simulink model "AUV_ControlsPreliminary"  (R2020b)
settings: Solver=ode23t  StartTime=0.0  StopTime=300  MaxStep=0.01  RelTol=1e-3  EnableMultiTasking=on
PreLoadFcn:
  | AUV_VehicleParameters;
  | Vehicle.Body.markeropacity = 0;
model workspace: external: MATLAB File AUV_DataFile_ORIG.m (data not in the file)
undefined symbols (not defined in the file or in its folder): Environment, Multibody, Newton, Raphson, smiData, X, x, Y, y, Z
libraries: sm_lib x3123, nesl_utility x51, sharedutil x8, pid_lib x6, AUVCustomPrimitives_Lib x4, shared6dof x1, aerolibasang x1, aerolibadyn x1, SignalEditorBlockLib x1
(part 2 of 62)

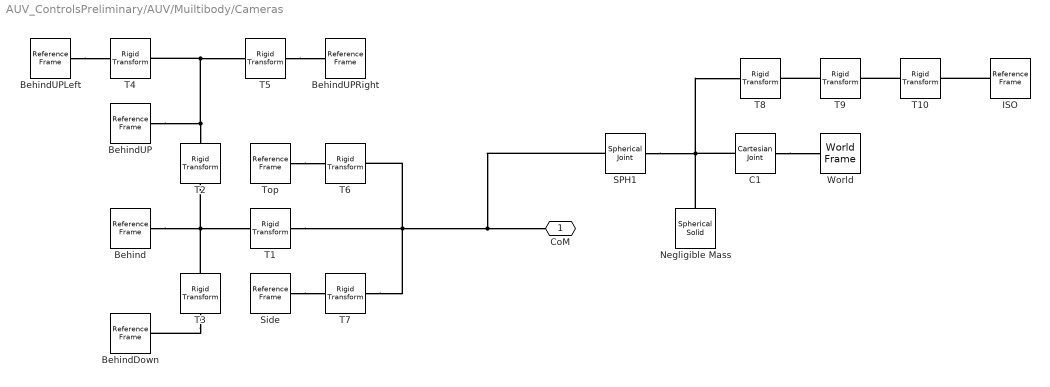
== system AUV_ControlsPreliminary/AUV/Muiltibody/Cameras ==
  Behind : sm_lib/Frames and Transforms/Reference Frame
  BehindDown : sm_lib/Frames and Transforms/Reference Frame
  BehindUP : sm_lib/Frames and Transforms/Reference Frame
  BehindUPLeft : sm_lib/Frames and Transforms/Reference Frame
  BehindUPRight : sm_lib/Frames and Transforms/Reference Frame
  C1 : sm_lib/Joints/Cartesian Joint  JointMode=Normal  SenseConstraintForce=off  SenseConstraintForceX=off  SenseConstraintForceY=off  SenseConstraintForceZ=off  SenseConstraintTorque=off  SenseConstraintTorqueX=off  SenseConstraintTorqueY=off  SenseConstraintTorqueZ=off  SenseTotalForce=off  SenseTotalForceX=off  SenseTotalForceY=off  SenseTotalForceZ=off  SenseTotalTorque=off  SenseTotalTorqueX=off  SenseTotalTorqueY=off  SenseTotalTorqueZ=off  CompositeWrenchDir=FollowerOnBase  CompositeWrenchFrame=BaseFrame  PxEquilibriumPosition=0  PxEquilibriumPositionUnits=m  PxSpringStiffness=0  PxSpringStiffnessUnits=N/m  PxDampingCoefficient=0  PxDampingCoefficientUnits=N/(m/s)  PxTorqueActuationMode=NoTorque  PxMotionActuationMode=ComputedMotion  PxSensePosition=off  PxSenseVelocity=off  PxSenseAcceleration=off  PxSenseTorqueForce=off  PxSenseLowerLimitTorqueForce=off  PxSenseUpperLimitTorqueForce=off  PxLowerLimitSpecify=off  PxLowerLimitBound=-1  PxLowerLimitBoundUnits=m  PxLowerLimitStiffness=1e6  PxLowerLimitStiffnessUnits=N/m  PxLowerLimitDamping=1e3  PxLowerLimitDampingUnits=N/(m/s)  PxLowerLimitTransitionRegionWidth=1e-4  PxLowerLimitTransitionRegionWidthUnits=m  PxUpperLimitSpecify=off  PxUpperLimitBound=1  PxUpperLimitBoundUnits=m  PxUpperLimitStiffness=1e6  PxUpperLimitStiffnessUnits=N/m  PxUpperLimitDamping=1e3  PxUpperLimitDampingUnits=N/(m/s)  PxUpperLimitTransitionRegionWidth=1e-4  PxUpperLimitTransitionRegionWidthUnits=m  PxPositionTargetSpecify=off  PxPositionTargetPriority=High  PxPositionTargetValue=0  PxPositionTargetValueUnits=m  PxVelocityTargetSpecify=off  PxVelocityTargetPriority=High  PxVelocityTargetValue=0  PxVelocityTargetValueUnits=m/s  PyEquilibriumPosition=0  PyEquilibriumPositionUnits=m  PySpringStiffness=0  PySpringStiffnessUnits=N/m  PyDampingCoefficient=0  PyDampingCoefficientUnits=N/(m/s)  PyTorqueActuationMode=NoTorque  PyMotionActuationMode=ComputedMotion  PySensePosition=off  PySenseVelocity=off  PySenseAcceleration=off  PySenseTorqueForce=off  PySenseLowerLimitTorqueForce=off  PySenseUpperLimitTorqueForce=off  PyLowerLimitSpecify=off  PyLowerLimitBound=-1  PyLowerLimitBoundUnits=m  PyLowerLimitStiffness=1e6  PyLowerLimitStiffnessUnits=N/m  PyLowerLimitDamping=1e3  PyLowerLimitDampingUnits=N/(m/s)  PyLowerLimitTransitionRegionWidth=1e-4  PyLowerLimitTransitionRegionWidthUnits=m  PyUpperLimitSpecify=off  PyUpperLimitBound=1  PyUpperLimitBoundUnits=m  PyUpperLimitStiffness=1e6  PyUpperLimitStiffnessUnits=N/m  PyUpperLimitDamping=1e3  PyUpperLimitDampingUnits=N/(m/s)  PyUpperLimitTransitionRegionWidth=1e-4  PyUpperLimitTransitionRegionWidthUnits=m  PyPositionTargetSpecify=off  PyPositionTargetPriority=High  PyPositionTargetValue=0  PyPositionTargetValueUnits=m  PyVelocityTargetSpecify=off  PyVelocityTargetPriority=High  PyVelocityTargetValue=0  PyVelocityTargetValueUnits=m/s  PzEquilibriumPosition=0  PzEquilibriumPositionUnits=m  PzSpringStiffness=0  PzSpringStiffnessUnits=N/m  PzDampingCoefficient=0  PzDampingCoefficientUnits=N/(m/s)  PzTorqueActuationMode=NoTorque  PzMotionActuationMode=ComputedMotion  PzSensePosition=off  PzSenseVelocity=off  PzSenseAcceleration=off  PzSenseTorqueForce=off  PzSenseLowerLimitTorqueForce=off  PzSenseUpperLimitTorqueForce=off  PzLowerLimitSpecify=off  PzLowerLimitBound=-1  PzLowerLimitBoundUnits=m  PzLowerLimitStiffness=1e6  PzLowerLimitStiffnessUnits=N/m  PzLowerLimitDamping=1e3  PzLowerLimitDampingUnits=N/(m/s)  PzLowerLimitTransitionRegionWidth=1e-4  PzLowerLimitTransitionRegionWidthUnits=m  PzUpperLimitSpecify=off  PzUpperLimitBound=1  PzUpperLimitBoundUnits=m  PzUpperLimitStiffness=1e6  PzUpperLimitStiffnessUnits=N/m  PzUpperLimitDamping=1e3  PzUpperLimitDampingUnits=N/(m/s)  PzUpperLimitTransitionRegionWidth=1e-4  PzUpperLimitTransitionRegionWidthUnits=m  PzPositionTargetSpecify=off  PzPositionTargetPriority=High  PzPositionTargetValue=0  PzPositionTargetValueUnits=m  PzVelocityTargetSpecify=off  PzVelocityTargetPriority=High  PzVelocityTargetValue=0  PzVelocityTargetValueUnits=m/s
  ISO : sm_lib/Frames and Transforms/Reference Frame
  Negligible Mass : sm_lib/Body Elements/Spherical Solid  GraphicAmbientColor=[0.15 0.15 0.15 1.0]  BasedOnType=Mass  CenterOfMass=[0 0 0]  CenterOfMassUnits=m  GraphicDiffuseColor=[0.5 0.5 0.5]  Density=1000  DensityUnits=kg/m^3  DoExposeReferenceFrame=on  GraphicEmissiveColor=[0.0 0.0 0.0 1.0]  ExportEntireGeometry=off  SerializedExposedGeometries=<ExposedGeometries/>  SerializedFrames=<Frames/>  MarkerShape=Sphere  MarkerSize=10  GraphicType=FromGeometry  InertiaType=CalculateFromGeometry  Mass=1e-6  MassUnits=kg  MomentsOfInertia=[1 1 1]  MomentsOfInertiaUnits=kg*m^2  GraphicOpacity=0  ProductsOfInertia=[0 0 0]  ProductsOfInertiaUnits=kg*m^2  GraphicShininess=75  GraphicSpecularColor=[0.5 0.5 0.5 1.0]  SphereRadius=1e-3  SphereRadiusUnits=m  GraphicVisPropType=SimpleVisualProperties
  SPH1 : sm_lib/Joints/Spherical Joint  JointMode=Normal  SenseConstraintForce=off  SenseConstraintForceX=off  SenseConstraintForceY=off  SenseConstraintForceZ=off  SenseConstraintTorque=off  SenseConstraintTorqueX=off  SenseConstraintTorqueY=off  SenseConstraintTorqueZ=off  SenseTotalForce=off  SenseTotalForceX=off  SenseTotalForceY=off  SenseTotalForceZ=off  SenseTotalTorque=off  SenseTotalTorqueX=off  SenseTotalTorqueY=off  SenseTotalTorqueZ=off  CompositeWrenchDir=FollowerOnBase  CompositeWrenchFrame=BaseFrame  DefPosRotationMethod=None  DefPosRotationAngleUnits=deg  DefPosRotationStandardAxis=+Z  DefPosRotationAngle=0.0  DefPosRotationArbitraryAxis=[0 0 1]  DefPosFollAlignAxisA=+X  DefPosBaseAlignAxisA=+Y  DefPosFollAlignAxisB=+Y  DefPosBaseAlignAxisB=+Z  DefPosRotationSequenceAxes=FollowerAxes  DefPosRotationSequence=XYX  DefPosRotationSequenceAngles=[0 0 0]  DefPosRotationSequenceAnglesUnits=deg  DefPosRotationMatrix=[1 0 0; 0 1 0; 0 0 1]  EqPosRotationMethod=None  EqPosRotationAngleUnits=deg  EqPosRotationStandardAxis=+Z  EqPosRotationAngle=0.0  EqPosRotationArbitraryAxis=[0 0 1]  EqPosFollAlignAxisA=+X  EqPosBaseAlignAxisA=+Y  EqPosFollAlignAxisB=+Y  EqPosBaseAlignAxisB=+Z  EqPosRotationSequenceAxes=FollowerAxes  EqPosRotationSequence=XYX  EqPosRotationSequenceAngles=[0 0 0]  EqPosRotationSequenceAnglesUnits=deg  EqPosRotationMatrix=[1 0 0; 0 1 0; 0 0 1]  SpringStiffness=0  SpringStiffnessUnits=N*m/deg  DampingCoefficient=0  DampingCoefficientUnits=N*m/(deg/s)  ActuateTorqueX=off  ActuateTorqueY=off  ActuateTorqueZ=off  ActuateTorque=off  TorqueActuationMode=NoTorque  MotionActuationMode=ComputedMotion  ActuationFrame=BaseFrame  SensePosition=off  SenseVelocityX=off  SenseVelocityY=off  SenseVelocityZ=off  SenseVelocity=off  SenseAccelerationX=off  SenseAccelerationY=off  SenseAccelerationZ=off  SenseAcceleration=off  SenseTorqueX=off  SenseTorqueY=off  SenseTorqueZ=off  SenseTorqueForce=off  SenseLowerLimitTorqueMag=off  SenseUpperLimitTorqueMag=off  SensingFrame=BaseFrame  LowerLimitSpecify=off  LowerLimitBound=15  LowerLimitBoundUnits=deg  LowerLimitStiffness=1e4  LowerLimitStiffnessUnits=N*m/deg  LowerLimitDamping=10  LowerLimitDampingUnits=N*m/(deg/s)  LowerLimitTransitionRegionWidth=0.1  LowerLimitTransitionRegionWidthUnits=deg  UpperLimitSpecify=off  UpperLimitBound=45  UpperLimitBoundUnits=deg  UpperLimitStiffness=1e4  UpperLimitStiffnessUnits=N*m/deg  UpperLimitDamping=10  UpperLimitDampingUnits=N*m/(deg/s)  UpperLimitTransitionRegionWidth=0.1  UpperLimitTransitionRegionWidthUnits=deg  PositionTargetRotationMethod=None  PositionTargetRotationAngleUnits=deg  PositionTargetRotationStandardAxis=+Z  PositionTargetRotationAngle=0.0  PositionTargetRotationArbitraryAxis=[0 0 1]  PositionTargetFollAlignAxisA=+X  PositionTargetBaseAlignAxisA=+Y  PositionTargetFollAlignAxisB=+Y  PositionTargetBaseAlignAxisB=+Z  PositionTargetRotationSequenceAxes=FollowerAxes  PositionTargetRotationSequence=XYX  PositionTargetRotationSequenceAngles=[0 0 0]  PositionTargetRotationSequenceAnglesUnits=deg  PositionTargetRotationMatrix=[1 0 0; 0 1 0; 0 0 1]  PositionTargetSpecify=off  PositionTargetPriority=High  VelocityTargetValue=[0 0 0]  VelocityTargetValueUnits=deg/s  VelocityTargetSpecify=off  VelocityTargetPriority=High  VelocityTargetInFollowerFrame=on
  Side : sm_lib/Frames and Transforms/Reference Frame
  T1 : sm_lib/Frames and Transforms/Rigid Transform  TranslationMethod=Cartesian  TranslationStandardOffset=0  TranslationLengthUnit=m  TranslationStandardAxis=+Z  TranslationCartesianOffset=[-3 0 0]  TranslationROffset=0  TranslationROffsetUnits=m  TranslationZOffset=0  TranslationZOffsetUnits=m  TranslationThetaOffset=0  TranslationThetaOffsetUnits=deg  RotationMethod=None  RotationAngleUnits=deg  RotationStandardAxis=+Z  RotationAngle=0.0  RotationArbitraryAxis=[0 0 1]  FollAlignAxisA=+X  BaseAlignAxisA=+Y  FollAlignAxisB=+Y  BaseAlignAxisB=+Z  RotationSequenceAxes=FollowerAxes  RotationSequence=XYX  RotationSequenceAngles=[0 0 0]  RotationSequenceAnglesUnits=deg  RotationMatrix=[1 0 0; 0 1 0; 0 0 1]
  T10 : sm_lib/Frames and Transforms/Rigid Transform  TranslationMethod=Cartesian  TranslationStandardOffset=0  TranslationLengthUnit=m  TranslationStandardAxis=+Z  TranslationCartesianOffset=[0 -1.5 0]  TranslationROffset=0  TranslationROffsetUnits=m  TranslationZOffset=0  TranslationZOffsetUnits=m  TranslationThetaOffset=0  TranslationThetaOffsetUnits=deg  RotationMethod=None  RotationAngleUnits=deg  RotationStandardAxis=+Z  RotationAngle=0.0  RotationArbitraryAxis=[0 0 1]  FollAlignAxisA=+X  BaseAlignAxisA=+Y  FollAlignAxisB=+Y  BaseAlignAxisB=+Z  RotationSequenceAxes=FollowerAxes  RotationSequence=XYX  RotationSequenceAngles=[0 0 0]  RotationSequenceAnglesUnits=deg  RotationMatrix=[1 0 0; 0 1 0; 0 0 1]
  T2 : sm_lib/Frames and Transforms/Rigid Transform  TranslationMethod=Cartesian  TranslationStandardOffset=0  TranslationLengthUnit=m  TranslationStandardAxis=+Z  TranslationCartesianOffset=[0 0 -3]  TranslationROffset=0  TranslationROffsetUnits=m  TranslationZOffset=0  TranslationZOffsetUnits=m  TranslationThetaOffset=0  TranslationThetaOffsetUnits=deg  RotationMethod=None  RotationAngleUnits=deg  RotationStandardAxis=+Z  RotationAngle=0.0  RotationArbitraryAxis=[0 0 1]  FollAlignAxisA=+X  BaseAlignAxisA=+Y  FollAlignAxisB=+Y  BaseAlignAxisB=+Z  RotationSequenceAxes=FollowerAxes  RotationSequence=XYX  RotationSequenceAngles=[0 0 0]  RotationSequenceAnglesUnits=deg  RotationMatrix=[1 0 0; 0 1 0; 0 0 1]
  T3 : sm_lib/Frames and Transforms/Rigid Transform  TranslationMethod=Cartesian  TranslationStandardOffset=0  TranslationLengthUnit=m  TranslationStandardAxis=+Z  TranslationCartesianOffset=[0 0 -3]  TranslationROffset=0  TranslationROffsetUnits=m  TranslationZOffset=0  TranslationZOffsetUnits=m  TranslationThetaOffset=0  TranslationThetaOffsetUnits=deg  RotationMethod=None  RotationAngleUnits=deg  RotationStandardAxis=+Z  RotationAngle=0.0  RotationArbitraryAxis=[0 0 1]  FollAlignAxisA=+X  BaseAlignAxisA=+Y  FollAlignAxisB=+Y  BaseAlignAxisB=+Z  RotationSequenceAxes=FollowerAxes  RotationSequence=XYX  RotationSequenceAngles=[0 0 0]  RotationSequenceAnglesUnits=deg  RotationMatrix=[1 0 0; 0 1 0; 0 0 1]
  T4 : sm_lib/Frames and Transforms/Rigid Transform  TranslationMethod=Cartesian  TranslationStandardOffset=0  TranslationLengthUnit=m  TranslationStandardAxis=+Z  TranslationCartesianOffset=[0 -2 0]  TranslationROffset=0  TranslationROffsetUnits=m  TranslationZOffset=0  TranslationZOffsetUnits=m  TranslationThetaOffset=0  TranslationThetaOffsetUnits=deg  RotationMethod=None  RotationAngleUnits=deg  RotationStandardAxis=+Z  RotationAngle=0.0  RotationArbitraryAxis=[0 0 1]  FollAlignAxisA=+X  BaseAlignAxisA=+Y  FollAlignAxisB=+Y  BaseAlignAxisB=+Z  RotationSequenceAxes=FollowerAxes  RotationSequence=XYX  RotationSequenceAngles=[0 0 0]  RotationSequenceAnglesUnits=deg  RotationMatrix=[1 0 0; 0 1 0; 0 0 1]
  T5 : sm_lib/Frames and Transforms/Rigid Transform  TranslationMethod=Cartesian  TranslationStandardOffset=0  TranslationLengthUnit=m  TranslationStandardAxis=+Z  TranslationCartesianOffset=[0 -2 0]  TranslationROffset=0  TranslationROffsetUnits=m  TranslationZOffset=0  TranslationZOffsetUnits=m  TranslationThetaOffset=0  TranslationThetaOffsetUnits=deg  RotationMethod=None  RotationAngleUnits=deg  RotationStandardAxis=+Z  RotationAngle=0.0  RotationArbitraryAxis=[0 0 1]  FollAlignAxisA=+X  BaseAlignAxisA=+Y  FollAlignAxisB=+Y  BaseAlignAxisB=+Z  RotationSequenceAxes=FollowerAxes  RotationSequence=XYX  RotationSequenceAngles=[0 0 0]  RotationSequenceAnglesUnits=deg  RotationMatrix=[1 0 0; 0 1 0; 0 0 1]
  T6 : sm_lib/Frames and Transforms/Rigid Transform  TranslationMethod=Cartesian  TranslationStandardOffset=0  TranslationLengthUnit=m  TranslationStandardAxis=+Z  TranslationCartesianOffset=[0 0 -3]  TranslationROffset=0  TranslationROffsetUnits=m  TranslationZOffset=0  TranslationZOffsetUnits=m  TranslationThetaOffset=0  TranslationThetaOffsetUnits=deg  RotationMethod=None  RotationAngleUnits=deg  RotationStandardAxis=+Z  RotationAngle=0.0  RotationArbitraryAxis=[0 0 1]  FollAlignAxisA=+X  BaseAlignAxisA=+Y  FollAlignAxisB=+Y  BaseAlignAxisB=+Z  RotationSequenceAxes=FollowerAxes  RotationSequence=XYX  RotationSequenceAngles=[0 0 0]  RotationSequenceAnglesUnits=deg  RotationMatrix=[1 0 0; 0 1 0; 0 0 1]
  T7 : sm_lib/Frames and Transforms/Rigid Transform  TranslationMethod=Cartesian  TranslationStandardOffset=0  TranslationLengthUnit=m  TranslationStandardAxis=+Z  TranslationCartesianOffset=[0 -3 0]  TranslationROffset=0  TranslationROffsetUnits=m  TranslationZOffset=0  TranslationZOffsetUnits=m  TranslationThetaOffset=0  TranslationThetaOffsetUnits=deg  RotationMethod=None  RotationAngleUnits=deg  RotationStandardAxis=+Z  RotationAngle=0.0  RotationArbitraryAxis=[0 0 1]  FollAlignAxisA=+X  BaseAlignAxisA=+Y  FollAlignAxisB=+Y  BaseAlignAxisB=+Z  RotationSequenceAxes=FollowerAxes  RotationSequence=XYX  RotationSequenceAngles=[0 0 0]  RotationSequenceAnglesUnits=deg  RotationMatrix=[1 0 0; 0 1 0; 0 0 1]
  T8 : sm_lib/Frames and Transforms/Rigid Transform  TranslationMethod=Cartesian  TranslationStandardOffset=0  TranslationLengthUnit=m  TranslationStandardAxis=+Z  TranslationCartesianOffset=[-2.5 0 0]  TranslationROffset=0  TranslationROffsetUnits=m  TranslationZOffset=0  TranslationZOffsetUnits=m  TranslationThetaOffset=0  TranslationThetaOffsetUnits=deg  RotationMethod=None  RotationAngleUnits=deg  RotationStandardAxis=+Z  RotationAngle=0.0  RotationArbitraryAxis=[0 0 1]  FollAlignAxisA=+X  BaseAlignAxisA=+Y  FollAlignAxisB=+Y  BaseAlignAxisB=+Z  RotationSequenceAxes=FollowerAxes  RotationSequence=XYX  RotationSequenceAngles=[0 0 0]  RotationSequenceAnglesUnits=deg  RotationMatrix=[1 0 0; 0 1 0; 0 0 1]
  T9 : sm_lib/Frames and Transforms/Rigid Transform  TranslationMethod=Cartesian  TranslationStandardOffset=0  TranslationLengthUnit=m  TranslationStandardAxis=+Z  TranslationCartesianOffset=[0 0 -2.5]  TranslationROffset=0  TranslationROffsetUnits=m  TranslationZOffset=0  TranslationZOffsetUnits=m  TranslationThetaOffset=0  TranslationThetaOffsetUnits=deg  RotationMethod=None  RotationAngleUnits=deg  RotationStandardAxis=+Z  RotationAngle=0.0  RotationArbitraryAxis=[0 0 1]  FollAlignAxisA=+X  BaseAlignAxisA=+Y  FollAlignAxisB=+Y  BaseAlignAxisB=+Z  RotationSequenceAxes=FollowerAxes  RotationSequence=XYX  RotationSequenceAngles=[0 0 0]  RotationSequenceAnglesUnits=deg  RotationMatrix=[1 0 0; 0 1 0; 0 0 1]
  Top : sm_lib/Frames and Transforms/Reference Frame
  World : sm_lib/Frames and Transforms/World Frame
  CoM : PMIOPort  Side=Right
  connections:
  T1/LConn1 -- T7/LConn1 -- SPH1/LConn1 -- CoM/RConn1 -- T6/LConn1
  Behind/RConn1 -- T3/RConn1 -- T2/LConn1 -- T1/RConn1
  BehindUP/RConn1 -- T2/RConn1 -- T5/RConn1 -- T4/LConn1
  T3/LConn1 -- BehindDown/RConn1
  BehindUPLeft/RConn1 -- T4/RConn1
  T5/LConn1 -- BehindUPRight/RConn1
  Top/RConn1 -- T6/RConn1
  Side/RConn1 -- T7/RConn1
  SPH1/RConn1 -- T8/LConn1 -- C1/LConn1 -- Negligible Mass/RConn1
  C1/RConn1 -- World/RConn1
  T9/LConn1 -- T8/RConn1
  T10/LConn1 -- T9/RConn1
  ISO/RConn1 -- T10/RConn1

== system AUV_ControlsPreliminary/AUV/Muiltibody/Hydro Forces & Moments ==
  Bus Element In : Inport  PortName=HydroForces  Element=Buoyancy.BForceZ
  Bus Element In1 : Inport  PortName=HydroForces  Element=LiftNDrag.LDForcesXYZ
  Bus Element In2 : Inport  PortName=HydroForces  Element=LiftNDrag.LDMomentsXYZ
  Bus Element In3 : Inport  PortName=HydroForces  Element=AddedMass.AMForcesXYZ
  Bus Element In4 : Inport  PortName=HydroForces  Element=AddedMass.AMMomentsXYZ
  Bus Element In5 : Inport  PortName=HydroForces  Element=AddedMass.CMomentsXYZ
  Bus Element In6 : Inport  PortName=HydroForces  Element=AddedMass.CForcesXYZ
  Added Mass Coriolis : Subsystem
  Added Mass Forces : Subsystem
  Buoyancy Force : Subsystem
  Lift and Drag Forces : Subsystem
  CoM : PMIOPort  Side=Right
  CoB : PMIOPort  Port=2  Side=Right
  wires:
  Bus Element In/1 -> Buoyancy Force/1(B)
  Bus Element In1/1 -> Lift and Drag Forces/1(Fxyz)
  Bus Element In2/1 -> Lift and Drag Forces/2(Mxyz)
  Bus Element In3/1 -> Added Mass Forces/1(Fxyz)
  Bus Element In4/1 -> Added Mass Forces/2(Mxyz)
  Bus Element In5/1 -> Added Mass Coriolis/2(Mxyz)
  Bus Element In6/1 -> Added Mass Coriolis/1(Fxyz)
  connections:
  CoB/RConn1 -- Buoyancy Force/RConn1
  Lift and Drag Forces/RConn1 -- Added Mass Coriolis/RConn1 -- Added Mass Forces/RConn1 -- CoM/RConn1

== system AUV_ControlsPreliminary/AUV/Muiltibody/World ==
  Mechanism Configuration : sm_lib/Utilities/Mechanism Configuration  UniformGravity=Constant  GravityVector=[0 0 Environment.gravity]  GravityVectorUnits=m/s^2  GravityUnits=m/s^2  LinearizationDelta=0.001  JointModeTransitionNonlinearIterations=2
  Sea Floor : Subsystem
  Solver Configuration : nesl_utility/Solver Configuration  PhysicalDomain=network_engine_domain  SubClassName=solver  LeftPortType=input  RightPortType=generic  Tones=[]  Harmonics=[]  SimulateNoise=off  Profile=off  UseLocalSampling=off  EnableSwitchedLinearOptims=on  FrequencyDomain=off  UseCCode=off  RelTol=0.001  AbsTol=1e-06  MinStep=1e-09  ToWorkspace=off  RevertToSquareIcSolve=off  NumHomotopyIterations=100  PhasorMode=off  PhasorModeNumHarmonics=1  DoDC=off  ResidualTolerance=1e-09  UseLocalSolver=off  LocalSolverChoice=NE_BACKWARD_EULER_ADVANCER  LocalSolverSampleTime=0.001  DoFixedCost=off  MaxNonlinIter=3  MaxModeIter=2  ComputeImpulses=off  ImpulseIterations=2  LinearAlgebra=Sparse  EquationFormulation=NE_TIME_EF  DelaysMemoryBudget=1024  AutomaticFiltering=on  FilteringTimeConstant=0.001  PartitionStorageMethod=AS_NEEDED  PartitionMemoryBudget=1024  PartitionMethod=FAST
  World Frame --> e NED : sm_lib/Frames and Transforms/World Frame
  W : PMIOPort  Side=Right
  connections:
  World Frame --> e NED/RConn1 -- W/RConn1 -- Sea Floor/LConn1 -- Mechanism Configuration/RConn1 -- Solver Configuration/RConn1

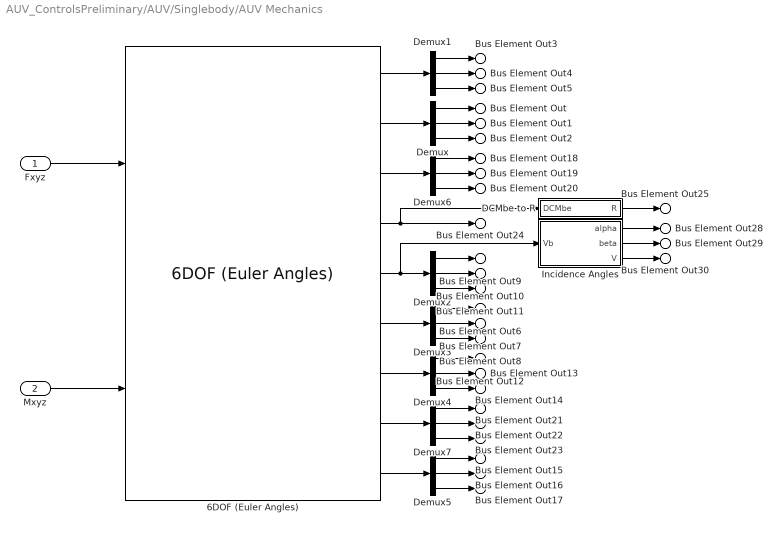
== system AUV_ControlsPreliminary/AUV/Singlebody/AUV Mechanics ==
  Fxyz : Inport
  Mxyz : Inport  Port=2
  6DOF (Euler Angles) : shared6dof/6DOF (Euler Angles)  units=Metric (MKS)  mtype=Fixed  rep=Euler Angles  xme_0=Vehicle.InitCond.position  Vm_0=Vehicle.InitCond.velocity  eul_0=Vehicle.InitCond.EulerXYZrad  pm_0=Vehicle.InitCond.rotrates  mass_0=Vehicle.Body.Full.mass  mass_e=0.5  mass_f=2.0  inertia=Vehicle.Body.Full.Inertia  inertia_e=eye(3)  inertia_f=2*eye(3)  k_quat=1.0  vre_flag=on  abi_flag=on  aMode=0  xme_statename=''  Vm_statename=''  eul_statename=''  quat_statename=''  pm_statename=''  mass_statename=''
      settings: SourceProductBaseCode=AE,PW,MT,UV,VE,VP
  DCMbe to R : Subsystem
  Demux{,1..7} (8 alike) : Demux  Outputs=3
  Incidence Angles : Subsystem
  Bus Element Out : Outport  PortName=CoM  Element=World.Xe.X
  Bus Element Out1 : Outport  PortName=CoM  Element=World.Xe.Y
  Bus Element Out2 : Outport  PortName=CoM  Element=World.Xe.Z
  Bus Element Out3 : Outport  PortName=CoM  Element=World.Ve.Vx
  Bus Element Out4 : Outport  PortName=CoM  Element=World.Ve.Vy
  Bus Element Out5 : Outport  PortName=CoM  Element=World.Ve.Vz
  Bus Element Out25 : Outport  PortName=CoM  Element=World.R
  Bus Element Out6 : Outport  PortName=CoM  Element=Body.wb.p
  Bus Element Out7 : Outport  PortName=CoM  Element=Body.wb.q
  Bus Element Out8 : Outport  PortName=CoM  Element=Body.wb.r
  Bus Element Out9 : Outport  PortName=CoM  Element=Body.Vb.u
  Bus Element Out10 : Outport  PortName=CoM  Element=Body.Vb.v
  Bus Element Out11 : Outport  PortName=CoM  Element=Body.Vb.w
  Bus Element Out12 : Outport  PortName=CoM  Element=Body.dwbdt.pdot
  Bus Element Out13 : Outport  PortName=CoM  Element=Body.dwbdt.qdot
  Bus Element Out14 : Outport  PortName=CoM  Element=Body.dwbdt.rdot
  Bus Element Out15 : Outport  PortName=CoM  Element=Body.Abe.ax
  Bus Element Out16 : Outport  PortName=CoM  Element=Body.Abe.ay
  Bus Element Out17 : Outport  PortName=CoM  Element=Body.Abe.az
  Bus Element Out18 : Outport  PortName=CoM  Element=Derived.Euler.phi
  Bus Element Out19 : Outport  PortName=CoM  Element=Derived.Euler.theta
  Bus Element Out20 : Outport  PortName=CoM  Element=Derived.Euler.psi
  Bus Element Out21 : Outport  PortName=CoM  Element=Derived.Body.Abb.Abbx
  Bus Element Out22 : Outport  PortName=CoM  Element=Derived.Body.Abb.Abby
  Bus Element Out23 : Outport  PortName=CoM  Element=Derived.Body.Abb.Abbz
  Bus Element Out28 : Outport  PortName=CoM  Element=Derived.Body.Incidences.alpha
  Bus Element Out29 : Outport  PortName=CoM  Element=Derived.Body.Incidences.beta
  Bus Element Out30 : Outport  PortName=CoM  Element=Derived.Body.V
  Bus Element Out24 : Outport  PortName=CoM  Element=Derived.World.DCMbe
  wires:
  Fxyz/1 -> 6DOF (Euler Angles)/1
  6DOF (Euler Angles)/2 -> Demux/1
  Mxyz/1 -> 6DOF (Euler Angles)/2
  Demux/2 -> Bus Element Out1/1
  Demux/1 -> Bus Element Out/1
  Demux/3 -> Bus Element Out2/1
  6DOF (Euler Angles)/1 -> Demux1/1
  Demux1/1 -> Bus Element Out3/1
  Demux1/2 -> Bus Element Out4/1
  Demux1/3 -> Bus Element Out5/1
  6DOF (Euler Angles)/5 -> Demux2/1, Incidence Angles/1(Vb)
  6DOF (Euler Angles)/6 -> Demux3/1
  Demux3/1 -> Bus Element Out6/1
  Demux3/2 -> Bus Element Out7/1
  Demux3/3 -> Bus Element Out8/1
  Demux2/1 -> Bus Element Out9/1
  Demux2/2 -> Bus Element Out10/1
  Demux2/3 -> Bus Element Out11/1
  6DOF (Euler Angles)/7 -> Demux4/1
  Demux4/1 -> Bus Element Out12/1
  Demux4/2 -> Bus Element Out13/1
  Demux4/3 -> Bus Element Out14/1
  6DOF (Euler Angles)/9 -> Demux5/1
  Demux5/1 -> Bus Element Out15/1
  Demux5/2 -> Bus Element Out16/1
  Demux5/3 -> Bus Element Out17/1
  6DOF (Euler Angles)/3 -> Demux6/1
  Demux6/1 -> Bus Element Out18/1
  Demux6/2 -> Bus Element Out19/1
  Demux6/3 -> Bus Element Out20/1
  6DOF (Euler Angles)/8 -> Demux7/1
  Demux7/1 -> Bus Element Out21/1
  Demux7/2 -> Bus Element Out22/1
  Demux7/3 -> Bus Element Out23/1
  6DOF (Euler Angles)/4 -> Bus Element Out24/1, DCMbe to R/1(DCMbe)
  Incidence Angles/1(alpha) -> Bus Element Out28/1
  Incidence Angles/2(beta) -> Bus Element Out29/1
  Incidence Angles/3(V) -> Bus Element Out30/1
  DCMbe to R/1(R) -> Bus Element Out25/1

== system AUV_ControlsPreliminary/AUV/Singlebody/Hydro Forces & Moments ==
  Bus Element In : Inport  PortName=HydroForces  Element=Buoyancy.BForceZ
  Bus Element In1 : Inport  PortName=HydroForces  Element=Weight.WForceZ
  Bus Element In3 : Inport  PortName=HydroForces  Element=AddedMass.AMForcesXYZ
  Bus Element In4 : Inport  PortName=HydroForces  Element=AddedMass.AMMomentsXYZ
  Bus Element In5 : Inport  PortName=HydroForces  Element=AddedMass.CForcesXYZ
  Bus Element In6 : Inport  PortName=HydroForces  Element=AddedMass.CMomentsXYZ
  Bus Element In7 : Inport  PortName=HydroForces  Element=LiftNDrag.LDForcesXYZ
  Bus Element In8 : Inport  PortName=HydroForces  Element=LiftNDrag.LDMomentsXYZ
  Bus Element In2 : Inport  Port=2  PortName=CoM  Element=Derived.World.DCMbe
  Added Mass Forces : Subsystem
  Hydrostatic Forces : Subsystem
  Lift and Drag Forces : Subsystem
  Sum : Sum  Inputs=+++
  Sum1 : Sum  Inputs=+++
  Fxyz : Outport
  Mxyz : Outport  Port=2
  wires:
  Bus Element In2/1 -> Hydrostatic Forces/1(DCM)
  Bus Element In/1 -> Hydrostatic Forces/2(Bz)
  Bus Element In1/1 -> Hydrostatic Forces/3(Wz)
  Bus Element In3/1 -> Added Mass Forces/1(AMFxyz)
  Bus Element In4/1 -> Added Mass Forces/2(AMMxyz)
  Bus Element In5/1 -> Added Mass Forces/3(AMCFxyz)
  Bus Element In6/1 -> Added Mass Forces/4(AMCMxyz)
  Bus Element In7/1 -> Lift and Drag Forces/1(LDFxyz)
  Bus Element In8/1 -> Lift and Drag Forces/2(LDMxyz)
  Lift and Drag Forces/1(Fxyz) -> Sum/2
  Sum/1 -> Fxyz/1
  Hydrostatic Forces/1(Fxyz) -> Sum/1
  Added Mass Forces/1(Fxyz) -> Sum/3
  Sum1/1 -> Mxyz/1
  Lift and Drag Forces/2(Mxyz) -> Sum1/2
  Hydrostatic Forces/2(Mxyz) -> Sum1/1
  Added Mass Forces/2(Mxyz) -> Sum1/3

== system AUV_ControlsPreliminary/AUV/Singlebody/Propellers & Thrusters ==
  Bus Element In : Inport  PortName=Actuators  Element=Propellers.PPf
  Bus Element In1 : Inport  PortName=Actuators  Element=Propellers.SPf
  Bus Element In2 : Inport  PortName=Actuators  Element=Thrusters.BHTf
  Bus Element In3 : Inport  PortName=Actuators  Element=Thrusters.BVTf
  Bus Element In4 : Inport  PortName=Actuators  Element=Thrusters.SHTf
  Bus Element In5 : Inport  PortName=Actuators  Element=Thrusters.SVTf
  Horizontal Tunnel Thrusters : Subsystem
  Main Propellers : Subsystem
  Sum : Sum  Inputs=+++
  Sum1 : Sum  Inputs=+++
  Vertical Tunnel Thrusters : Subsystem
  Fxyz : Outport
  Mxyz : Outport  Port=2
  wires:
  Bus Element In1/1 -> Main Propellers/1(SPf)
  Bus Element In/1 -> Main Propellers/2(PPf)
  Bus Element In3/1 -> Vertical Tunnel Thrusters/1(BVTf)
  Bus Element In5/1 -> Vertical Tunnel Thrusters/2(SVTf)
  Bus Element In2/1 -> Horizontal Tunnel Thrusters/1(BHTf)
  Bus Element In4/1 -> Horizontal Tunnel Thrusters/2(SHTf)
  Horizontal Tunnel Thrusters/1(Fxyz) -> Sum/2
  Sum/1 -> Fxyz/1
  Main Propellers/1(Fxyz) -> Sum/1
  Vertical Tunnel Thrusters/1(Fxyz) -> Sum/3
  Sum1/1 -> Mxyz/1
  Horizontal Tunnel Thrusters/2(Mxyz) -> Sum1/2
  Main Propellers/2(Mxyz) -> Sum1/1
  Vertical Tunnel Thrusters/2(Mxyz) -> Sum1/3

== system AUV_ControlsPreliminary/Dive Controls/Thrust Controls/Depth and Pitch Control ==
  note: NOTE: Vehicle depth is indirectly controlled by the pitch angle which is regulated by the vertical thrusters ONLY
  PPf : Inport
  SPf : Inport  Port=2
  ZRef : Inport  Port=3
  Z : Inport  Port=4
  theta : Inport  Port=5
  Gain2 : Gain  Gain=-1
  Main Propellers Thrust Offset Compensation : Subsystem
  PDtheta : pid_lib/PID Controller  Controller=PD  Form=Parallel  TimeDomain=Continuous-time  UseExternalTs=off  SampleTime=-1  IntegratorMethod=Forward Euler  FilterMethod=Forward Euler  ControllerParametersSource=internal  P=-2023.58  I=1  D=-2454.43  UseFilter=on  N=3588.47  TunerSelectOption=Transfer Function Based (PID Tuner App)  InitialConditionSource=internal  InitialConditionForIntegrator=0  InitialConditionForFilter=0  DifferentiatorICPrevScaledInput=0  ExternalReset=none  TrackingMode=off  Kt=1  LimitOutput=off  SatLimitsSource=internal  UpperSaturationLimit=inf  LowerSaturationLimit=-inf  LinearizeAsGain=on  AntiWindupMode=none  Kb=1  POutMin=[]  POutMax=[]  IOutMin=[]  IOutMax=[]  DOutMin=[]  DOutMax=[]  NOutMin=[]  NOutMax=[]  SumOutMin=[]  SumOutMax=[]  SaturationOutMin=[]  SaturationOutMax=[]  PParamMin=[]  PParamMax=[]  IParamMin=[]  IParamMax=[]  DParamMin=[]  DParamMax=[]  NParamMin=[]  NParamMax=[]  KbParamMin=[]  KbParamMax=[]  KtParamMin=[]  KtParamMax=[]  KbOutMin=[]  KbOutMax=[]  KtOutMin=[]  KtOutMax=[]  IntegratorOutMin=[]  IntegratorOutMax=[]  FilterOutMin=[]  FilterOutMax=[]  SumI1OutMin=[]  SumI1OutMax=[]  SumI2OutMin=[]  SumI2OutMax=[]  SumI3OutMin=[]  SumI3OutMax=[]  SumI4OutMin=[]  SumI4OutMax=[]  SumDOutMin=[]  SumDOutMax=[]  DifferentiatorOutMin=[]  DifferentiatorOutMax=[]  FilterDiffOutCoefMin=[]  FilterDiffOutCoefMax=[]  ReciprocalOutMin=[]  ReciprocalOutMax=[]  SumDenOutMin=[]  SumDenOutMax=[]  SumNumOutMin=[]  SumNumOutMax=[]  DivideOutMin=[]  DivideOutMax=[]  UdiffTsProdOutMin=[]  UdiffTsProdOutMax=[]  NTsProdOutMin=[]  NTsProdOutMax=[]  UintegralTsProdOutMin=[]  UintegralTsProdOutMax=[]  UngainTsProdOutMin=[]  UngainTsProdOutMax=[]  IntegratorContinuousStateAttributes=''  IntegratorStateMustResolveToSignalObject=off  IntegratorRTWStateStorageClass=Auto  FilterContinuousStateAttributes=''  FilterStateMustResolveToSignalObject=off  FilterRTWStateStorageClass=Auto  ParallelPVariant=InternalParameters  IdealPVariant=Disabled  IVariant=Disabled  DVariant=InternalParameters  IntegratorVariant=Disabled  SatVariant=Disabled  AWVariant=Disabled  PCopyVariant=Disabled  TRVariant=Disabled  FdbkBlocksVariant=Forward  IdealPFdbkVariant=Disabled  SatFdbkVariant=Disabled  DerivativeFilterVariant=ContFilter  NVariant=InternalParameters  NCopyVariant=Disabled  FilterICVariant=InternalICsFilter  IntegratorICVariant=Disabled  ExternalResetVariant=Disabled  TRSumVariant=Passthrough  SumFdbkVariant=Disabled  SumVariant=Sum_PD  TsampFilterVariant=InternalTs  TsampNgainVariant=Passthrough  TsampIntegralVariant=Disabled_SignalSpec  ExternalSaturationOutDataTypeStr=Inherit: Same as second input
  PIZ : pid_lib/PID Controller  Controller=PI  Form=Parallel  TimeDomain=Continuous-time  UseExternalTs=off  SampleTime=-1  IntegratorMethod=Forward Euler  FilterMethod=Forward Euler  ControllerParametersSource=internal  P=-0.25  I=-0.001  D=0  UseFilter=on  N=100  TunerSelectOption=Transfer Function Based (PID Tuner App)  InitialConditionSource=internal  InitialConditionForIntegrator=0  InitialConditionForFilter=0  DifferentiatorICPrevScaledInput=0  ExternalReset=none  TrackingMode=off  Kt=1  LimitOutput=off  SatLimitsSource=internal  UpperSaturationLimit=inf  LowerSaturationLimit=-inf  LinearizeAsGain=on  AntiWindupMode=none  Kb=1  POutMin=[]  POutMax=[]  IOutMin=[]  IOutMax=[]  DOutMin=[]  DOutMax=[]  NOutMin=[]  NOutMax=[]  SumOutMin=[]  SumOutMax=[]  SaturationOutMin=[]  SaturationOutMax=[]  PParamMin=[]  PParamMax=[]  IParamMin=[]  IParamMax=[]  DParamMin=[]  DParamMax=[]  NParamMin=[]  NParamMax=[]  KbParamMin=[]  KbParamMax=[]  KtParamMin=[]  KtParamMax=[]  KbOutMin=[]  KbOutMax=[]  KtOutMin=[]  KtOutMax=[]  IntegratorOutMin=[]  IntegratorOutMax=[]  FilterOutMin=[]  FilterOutMax=[]  SumI1OutMin=[]  SumI1OutMax=[]  SumI2OutMin=[]  SumI2OutMax=[]  SumI3OutMin=[]  SumI3OutMax=[]  SumI4OutMin=[]  SumI4OutMax=[]  SumDOutMin=[]  SumDOutMax=[]  DifferentiatorOutMin=[]  DifferentiatorOutMax=[]  FilterDiffOutCoefMin=[]  FilterDiffOutCoefMax=[]  ReciprocalOutMin=[]  ReciprocalOutMax=[]  SumDenOutMin=[]  SumDenOutMax=[]  SumNumOutMin=[]  SumNumOutMax=[]  DivideOutMin=[]  DivideOutMax=[]  UdiffTsProdOutMin=[]  UdiffTsProdOutMax=[]  NTsProdOutMin=[]  NTsProdOutMax=[]  UintegralTsProdOutMin=[]  UintegralTsProdOutMax=[]  UngainTsProdOutMin=[]  UngainTsProdOutMax=[]  IntegratorContinuousStateAttributes=''  IntegratorStateMustResolveToSignalObject=off  IntegratorRTWStateStorageClass=Auto  FilterContinuousStateAttributes=''  FilterStateMustResolveToSignalObject=off  FilterRTWStateStorageClass=Auto  ParallelPVariant=InternalParameters  IdealPVariant=Disabled  IVariant=InternalParameters  DVariant=Disabled  IntegratorVariant=Continuous  SatVariant=Disabled  AWVariant=Passthrough  PCopyVariant=Disabled  TRVariant=Disabled  FdbkBlocksVariant=Forward  IdealPFdbkVariant=Disabled  SatFdbkVariant=Disabled  DerivativeFilterVariant=Disabled  NVariant=Disabled  NCopyVariant=Disabled_SignalSpec  FilterICVariant=Disabled  IntegratorICVariant=InternalICs  ExternalResetVariant=Disabled  TRSumVariant=Passthrough  SumFdbkVariant=Disabled  SumVariant=Sum_PI  TsampFilterVariant=InternalTs  TsampNgainVariant=Passthrough  TsampIntegralVariant=Passthrough  ExternalSaturationOutDataTypeStr=Inherit: Same as second input
  Sum : Sum  Inputs=|+-
  Sum1 : Sum  Inputs=++|
  Sum2 : Sum  Inputs=|+-
  BVTfcmd : Outport
  SVTfcmd : Outport  Port=2
  wires:
  PPf/1 -> Main Propellers Thrust Offset Compensation/1(PPf)
  SPf/1 -> Main Propellers Thrust Offset Compensation/2(SPf)
  Gain2/1 -> SVTfcmd/1
  theta/1 -> Sum/2
  Sum/1 -> PDtheta/1
  PDtheta/1 -> Sum1/2
  Sum1/1 -> Gain2/1, BVTfcmd/1
  ZRef/1 -> Sum2/1
  Z/1 -> Sum2/2
  Sum2/1 -> PIZ/1
  PIZ/1 -> Sum/1
  Main Propellers Thrust Offset Compensation/1(VTf) -> Sum1/1

== system AUV_ControlsPreliminary/Dive Controls/Thrust Controls/Heading and Yaw Control ==
  note: NOTE: Vehicle heading is regulated by the horizontal thrusters ONLY
  v : Inport
  psiRef : Inport  Port=2
  pqr : Inport  Port=3
  phithetapsi : Inport  Port=4
  Bus Selector : BusSelector  OutputSignals=psi
  Gain : Gain  Gain=-1
  PIDpsi : pid_lib/PID Controller  Controller=PID  Form=Parallel  TimeDomain=Continuous-time  UseExternalTs=off  SampleTime=-1  IntegratorMethod=Forward Euler  FilterMethod=Forward Euler  ControllerParametersSource=internal  P=564.0086345182  I=63718.733398644  D=1.06148768314347  UseFilter=on  N=71769.5968954127  TunerSelectOption=Transfer Function Based (PID Tuner App)  InitialConditionSource=internal  InitialConditionForIntegrator=0  InitialConditionForFilter=0  DifferentiatorICPrevScaledInput=0  ExternalReset=none  TrackingMode=off  Kt=1  LimitOutput=off  SatLimitsSource=internal  UpperSaturationLimit=inf  LowerSaturationLimit=-inf  LinearizeAsGain=on  AntiWindupMode=none  Kb=1  POutMin=[]  POutMax=[]  IOutMin=[]  IOutMax=[]  DOutMin=[]  DOutMax=[]  NOutMin=[]  NOutMax=[]  SumOutMin=[]  SumOutMax=[]  SaturationOutMin=[]  SaturationOutMax=[]  PParamMin=[]  PParamMax=[]  IParamMin=[]  IParamMax=[]  DParamMin=[]  DParamMax=[]  NParamMin=[]  NParamMax=[]  KbParamMin=[]  KbParamMax=[]  KtParamMin=[]  KtParamMax=[]  KbOutMin=[]  KbOutMax=[]  KtOutMin=[]  KtOutMax=[]  IntegratorOutMin=[]  IntegratorOutMax=[]  FilterOutMin=[]  FilterOutMax=[]  SumI1OutMin=[]  SumI1OutMax=[]  SumI2OutMin=[]  SumI2OutMax=[]  SumI3OutMin=[]  SumI3OutMax=[]  SumI4OutMin=[]  SumI4OutMax=[]  SumDOutMin=[]  SumDOutMax=[]  DifferentiatorOutMin=[]  DifferentiatorOutMax=[]  FilterDiffOutCoefMin=[]  FilterDiffOutCoefMax=[]  ReciprocalOutMin=[]  ReciprocalOutMax=[]  SumDenOutMin=[]  SumDenOutMax=[]  SumNumOutMin=[]  SumNumOutMax=[]  DivideOutMin=[]  DivideOutMax=[]  UdiffTsProdOutMin=[]  UdiffTsProdOutMax=[]  NTsProdOutMin=[]  NTsProdOutMax=[]  UintegralTsProdOutMin=[]  UintegralTsProdOutMax=[]  UngainTsProdOutMin=[]  UngainTsProdOutMax=[]  IntegratorContinuousStateAttributes=''  IntegratorStateMustResolveToSignalObject=off  IntegratorRTWStateStorageClass=Auto  FilterContinuousStateAttributes=''  FilterStateMustResolveToSignalObject=off  FilterRTWStateStorageClass=Auto  ParallelPVariant=InternalParameters  IdealPVariant=Disabled  IVariant=InternalParameters  DVariant=InternalParameters  IntegratorVariant=Continuous  SatVariant=Disabled  AWVariant=Passthrough  PCopyVariant=Disabled  TRVariant=Disabled  FdbkBlocksVariant=Forward  IdealPFdbkVariant=Disabled  SatFdbkVariant=Disabled  DerivativeFilterVariant=ContFilter  NVariant=InternalParameters  NCopyVariant=Disabled  FilterICVariant=InternalICsFilter  IntegratorICVariant=InternalICs  ExternalResetVariant=Disabled  TRSumVariant=Passthrough  SumFdbkVariant=Disabled  SumVariant=Sum_PID  TsampFilterVariant=InternalTs  TsampNgainVariant=Passthrough  TsampIntegralVariant=Passthrough  ExternalSaturationOutDataTypeStr=Inherit: Same as second input
  PIDpsidot : pid_lib/PID Controller  Controller=PID  Form=Parallel  TimeDomain=Continuous-time  UseExternalTs=off  SampleTime=-1  IntegratorMethod=Forward Euler  FilterMethod=Forward Euler  ControllerParametersSource=internal  P=36876.176480623  I=4618545.3057506  D=-22.9389890340326  UseFilter=on  N=628  TunerSelectOption=Transfer Function Based (PID Tuner App)  InitialConditionSource=internal  InitialConditionForIntegrator=0  InitialConditionForFilter=0  DifferentiatorICPrevScaledInput=0  ExternalReset=none  TrackingMode=off  Kt=1  LimitOutput=off  SatLimitsSource=internal  UpperSaturationLimit=inf  LowerSaturationLimit=-inf  LinearizeAsGain=on  AntiWindupMode=none  Kb=1  POutMin=[]  POutMax=[]  IOutMin=[]  IOutMax=[]  DOutMin=[]  DOutMax=[]  NOutMin=[]  NOutMax=[]  SumOutMin=[]  SumOutMax=[]  SaturationOutMin=[]  SaturationOutMax=[]  PParamMin=[]  PParamMax=[]  IParamMin=[]  IParamMax=[]  DParamMin=[]  DParamMax=[]  NParamMin=[]  NParamMax=[]  KbParamMin=[]  KbParamMax=[]  KtParamMin=[]  KtParamMax=[]  KbOutMin=[]  KbOutMax=[]  KtOutMin=[]  KtOutMax=[]  IntegratorOutMin=[]  IntegratorOutMax=[]  FilterOutMin=[]  FilterOutMax=[]  SumI1OutMin=[]  SumI1OutMax=[]  SumI2OutMin=[]  SumI2OutMax=[]  SumI3OutMin=[]  SumI3OutMax=[]  SumI4OutMin=[]  SumI4OutMax=[]  SumDOutMin=[]  SumDOutMax=[]  DifferentiatorOutMin=[]  DifferentiatorOutMax=[]  FilterDiffOutCoefMin=[]  FilterDiffOutCoefMax=[]  ReciprocalOutMin=[]  ReciprocalOutMax=[]  SumDenOutMin=[]  SumDenOutMax=[]  SumNumOutMin=[]  SumNumOutMax=[]  DivideOutMin=[]  DivideOutMax=[]  UdiffTsProdOutMin=[]  UdiffTsProdOutMax=[]  NTsProdOutMin=[]  NTsProdOutMax=[]  UintegralTsProdOutMin=[]  UintegralTsProdOutMax=[]  UngainTsProdOutMin=[]  UngainTsProdOutMax=[]  IntegratorContinuousStateAttributes=''  IntegratorStateMustResolveToSignalObject=off  IntegratorRTWStateStorageClass=Auto  FilterContinuousStateAttributes=''  FilterStateMustResolveToSignalObject=off  FilterRTWStateStorageClass=Auto  ParallelPVariant=InternalParameters  IdealPVariant=Disabled  IVariant=InternalParameters  DVariant=InternalParameters  IntegratorVariant=Continuous  SatVariant=Disabled  AWVariant=Passthrough  PCopyVariant=Disabled  TRVariant=Disabled  FdbkBlocksVariant=Forward  IdealPFdbkVariant=Disabled  SatFdbkVariant=Disabled  DerivativeFilterVariant=ContFilter  NVariant=InternalParameters  NCopyVariant=Disabled  FilterICVariant=InternalICsFilter  IntegratorICVariant=InternalICs  ExternalResetVariant=Disabled  TRSumVariant=Passthrough  SumFdbkVariant=Disabled  SumVariant=Sum_PID  TsampFilterVariant=InternalTs  TsampNgainVariant=Passthrough  TsampIntegralVariant=Passthrough  ExternalSaturationOutDataTypeStr=Inherit: Same as second input
  Sum : Sum  Inputs=-+|
  Sum1 : Sum  Inputs=-+|
  Sum2 : Sum  Inputs=++|
  Sum3 : Sum  Inputs=++|
  psidot : Subsystem
  side slip compensation : Subsystem
  BHTfcmd : Outport
  SHTfcmd : Outport  Port=2
  wires:
  pqr/1 -> psidot/1(pqr)
  phithetapsi/1 -> psidot/2(phithetapsi), Bus Selector/1
  psidot/1(psid) -> Sum/1
  Sum/1 -> PIDpsidot/1
  PIDpsidot/1 -> Gain/1, Sum2/2
  Sum1/1 -> PIDpsi/1
  PIDpsi/1 -> Sum/2
  Bus Selector/1 -> Sum1/1  "<psi>"
  psiRef/1 -> Sum1/2
  Sum2/1 -> BHTfcmd/1
  Gain/1 -> Sum3/2
  Sum3/1 -> SHTfcmd/1
  v/1 -> side slip compensation/1(v)
  side slip compensation/1(BHTf) -> Sum2/1
  side slip compensation/2(SHTf) -> Sum3/1

== system AUV_ControlsPreliminary/Dive Controls/Thrust Controls/Longitudinal Speed (Surge) Control ==
  note: NOTE: Vehicle longitudinal speed is regulated by the main propellers ONLY
  uRef : Inport
  u : Inport  Port=2
  PIu : pid_lib/PID Controller  Controller=PI  Form=Parallel  TimeDomain=Continuous-time  UseExternalTs=off  SampleTime=-1  IntegratorMethod=Forward Euler  FilterMethod=Forward Euler  ControllerParametersSource=internal  P=78.8975  I=17.2606  D=0  UseFilter=on  N=100  TunerSelectOption=Transfer Function Based (PID Tuner App)  InitialConditionSource=internal  InitialConditionForIntegrator=0  InitialConditionForFilter=0  DifferentiatorICPrevScaledInput=0  ExternalReset=none  TrackingMode=off  Kt=1  LimitOutput=off  SatLimitsSource=internal  UpperSaturationLimit=inf  LowerSaturationLimit=-inf  LinearizeAsGain=on  AntiWindupMode=none  Kb=1  POutMin=[]  POutMax=[]  IOutMin=[]  IOutMax=[]  DOutMin=[]  DOutMax=[]  NOutMin=[]  NOutMax=[]  SumOutMin=[]  SumOutMax=[]  SaturationOutMin=[]  SaturationOutMax=[]  PParamMin=[]  PParamMax=[]  IParamMin=[]  IParamMax=[]  DParamMin=[]  DParamMax=[]  NParamMin=[]  NParamMax=[]  KbParamMin=[]  KbParamMax=[]  KtParamMin=[]  KtParamMax=[]  KbOutMin=[]  KbOutMax=[]  KtOutMin=[]  KtOutMax=[]  IntegratorOutMin=[]  IntegratorOutMax=[]  FilterOutMin=[]  FilterOutMax=[]  SumI1OutMin=[]  SumI1OutMax=[]  SumI2OutMin=[]  SumI2OutMax=[]  SumI3OutMin=[]  SumI3OutMax=[]  SumI4OutMin=[]  SumI4OutMax=[]  SumDOutMin=[]  SumDOutMax=[]  DifferentiatorOutMin=[]  DifferentiatorOutMax=[]  FilterDiffOutCoefMin=[]  FilterDiffOutCoefMax=[]  ReciprocalOutMin=[]  ReciprocalOutMax=[]  SumDenOutMin=[]  SumDenOutMax=[]  SumNumOutMin=[]  SumNumOutMax=[]  DivideOutMin=[]  DivideOutMax=[]  UdiffTsProdOutMin=[]  UdiffTsProdOutMax=[]  NTsProdOutMin=[]  NTsProdOutMax=[]  UintegralTsProdOutMin=[]  UintegralTsProdOutMax=[]  UngainTsProdOutMin=[]  UngainTsProdOutMax=[]  IntegratorContinuousStateAttributes=''  IntegratorStateMustResolveToSignalObject=off  IntegratorRTWStateStorageClass=Auto  FilterContinuousStateAttributes=''  FilterStateMustResolveToSignalObject=off  FilterRTWStateStorageClass=Auto  ParallelPVariant=InternalParameters  IdealPVariant=Disabled  IVariant=InternalParameters  DVariant=Disabled  IntegratorVariant=Continuous  SatVariant=Disabled  AWVariant=Passthrough  PCopyVariant=Disabled  TRVariant=Disabled  FdbkBlocksVariant=Forward  IdealPFdbkVariant=Disabled  SatFdbkVariant=Disabled  DerivativeFilterVariant=Disabled  NVariant=Disabled  NCopyVariant=Disabled_SignalSpec  FilterICVariant=Disabled  IntegratorICVariant=InternalICs  ExternalResetVariant=Disabled  TRSumVariant=Passthrough  SumFdbkVariant=Disabled  SumVariant=Sum_PI  TsampFilterVariant=InternalTs  TsampNgainVariant=Passthrough  TsampIntegralVariant=Passthrough  ExternalSaturationOutDataTypeStr=Inherit: Same as second input
  Sum : Sum  Inputs=|+-
  PPfcmd : Outport
  SPfcmd : Outport  Port=2
  wires:
  Sum/1 -> PIu/1
  PIu/1 -> PPfcmd/1, SPfcmd/1
  u/1 -> Sum/2
  uRef/1 -> Sum/1

== system AUV_ControlsPreliminary/Hydrostatic & Hydrodynamic Effects/Added Mass Forces/Added Mass ==
  note: NOTE:
      | The forces due to added mass will me applied as external
      | forces, so they will oppose the direction of the accelerations
      |
      | $M_{rb}\dot{\nu}+C_{rb}(\nu)\nu= F_{propulsion} - M_a\dot{\nu}-C_a(\nu)\nu-D(\nu)\nu$
  Ma : Inport
  Abb : Inport  Port=2
  dwbdt : Inport  Port=3
  Demux : Demux  Outputs=[3,3]
  Gain : Gain  Gain=-1
  LPfilter : Subsystem
  Ma*[Abb,dwbdt]' : Product  Multiplication=Matrix(*)
  "[Abb,dwbdt]'" : Concatenate  Mode=Multidimensional array
  Fxyz : Outport
  Mxyz : Outport  Port=2
  wires:
  dwbdt/1 -> "[Abb,dwbdt]'"/2
  "[Abb,dwbdt]'"/1 -> Ma*[Abb,dwbdt]'/2
  Demux/2 -> Mxyz/1
  Ma/1 -> Ma*[Abb,dwbdt]'/1
  Abb/1 -> "[Abb,dwbdt]'"/1
  Demux/1 -> Fxyz/1
  Ma*[Abb,dwbdt]'/1 -> LPfilter/1(in)
  LPfilter/1(out) -> Gain/1
  Gain/1 -> Demux/1

== system AUV_ControlsPreliminary/Hydrostatic & Hydrodynamic Effects/Added Mass Forces/Coriolis ==
  note: Coriolis matrix
  note: NOTE:
      | It is important to mention that the coriolis matrix due to added mass
      | computed here includes the de-stabilizing Munk-moment .
      | This moment acts to turn the vehicle perpendicular to the flow, and it
      | is most dominant for slender body vehicles in pitch and yaw when the
      | lateral velocities are non-zero.
      | This de-stabilizing effect will need to be accounted for in the design
      | of the control algorithm.
  Vb : Inport
  wb : Inport  Port=2
  Ma : Inport  Port=3
  Ca(V) : Subsystem
  Ca(V)*[Vb,wb]' : Product  Multiplication=Matrix(*)
  Demux : Demux  Outputs=6
  Demux1 : Demux  Outputs=[3,3]
  Gain : Gain  Gain=-1
  Ma*[Vb,wb]' : Product  Multiplication=Matrix(*)
  "[Vb,wb]'" : Concatenate  Mode=Multidimensional array
  Fxyz : Outport
  Mxyz : Outport  Port=2
  wires:
  Ma/1 -> Ma*[Vb,wb]'/1
  Vb/1 -> "[Vb,wb]'"/1
  wb/1 -> "[Vb,wb]'"/2
  "[Vb,wb]'"/1 -> Ca(V)*[Vb,wb]'/2, Ma*[Vb,wb]'/2
  Ma*[Vb,wb]'/1 -> Demux/1
  Demux/1 -> Ca(V)/1(a1)  "a1"
  Demux/2 -> Ca(V)/2(a2)  "a2"
  Demux/3 -> Ca(V)/3(a3)  "a3"
  Demux/4 -> Ca(V)/4(b1)  "b1"
  Demux/5 -> Ca(V)/5(b2)  "b2"
  Demux/6 -> Ca(V)/6(b3)  "b3"
  Ca(V)/1(Ca(V)) -> Ca(V)*[Vb,wb]'/1
  Ca(V)*[Vb,wb]'/1 -> Gain/1
  Demux1/1 -> Fxyz/1
  Demux1/2 -> Mxyz/1
  Gain/1 -> Demux1/1

== system AUV_ControlsPreliminary/Hydrostatic & Hydrodynamic Effects/Lift and Drag Forces/Hydrodynamic Coefficients ==
  alpha,beta : Inport
  wb : Inport  Port=2
  Vb : Inport  Port=3
  Body Rate Damping : Subsystem
  Demux : Demux  Outputs=2
  Drag and Lift Coefficients : Subsystem
  Sum : Sum  Inputs=++|
  rad to deg : UnitConversion
  Coeff : Outport
  wires:
  alpha,beta/1 -> rad to deg/1
  rad to deg/1 -> Demux/1
  Demux/1 -> Body Rate Damping/3(alpha), Drag and Lift Coefficients/1(alpha)
  Demux/2 -> Drag and Lift Coefficients/2(beta)
  Vb/1 -> Body Rate Damping/1(Vb)
  wb/1 -> Body Rate Damping/2(pqr)
  Drag and Lift Coefficients/1(coeff) -> Sum/2
  Body Rate Damping/1(coeff) -> Sum/1
  Sum/1 -> Coeff/1
